simulink model "pwm_motor"  (R2021b)
settings: Solver=VariableStepAuto  StartTime=0.0  StopTime=1  RelTol=1e-3
undefined symbols (not defined in the file or in its folder): J, km, L, R, Vmax
libraries: simulink x2
settings Model: Creator=cirie  LastModifiedBy=cirie

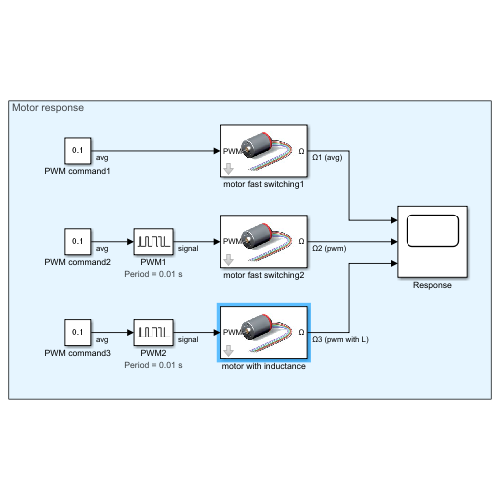
[thumbnail: Simulink's stored preview of the top-level diagram]
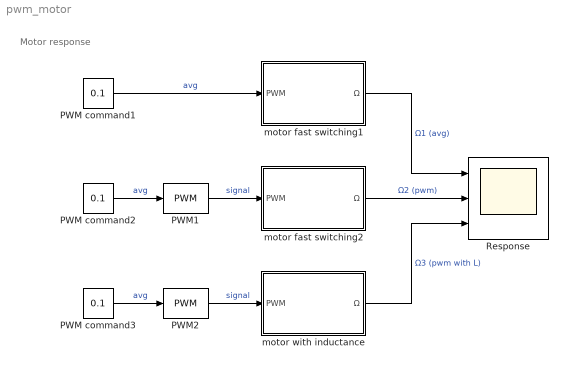
== system pwm_motor ==
  note: Motor response
  PWM command1 : Constant  Value=0.1
  PWM command2 : Constant  Value=0.1
  PWM command3 : Constant  Value=0.1
  PWM1 : simulink/Discontinuities/PWM  DisableCoverage=on  Period=0.01  DisallowZeroDutyCycle=off  RunAtFixedTimeIntervals=off  SampleTime=0.01
      settings: AttributesFormatString=Period = %<Period> s
  PWM2 : simulink/Discontinuities/PWM  DisableCoverage=on  Period=0.01  DisallowZeroDutyCycle=off  RunAtFixedTimeIntervals=off  SampleTime=0.01
      settings: AttributesFormatString=Period = %<Period> s
  Response : Scope  NumInputPorts=3
  motor fast switching1 : Subsystem  mask(DC Motor){J=J, km=km, R=R, Vmax=Vmax}
      mask prompts: J "Inertia, J [kgm^2]"; km "Motor constant, km [V*s/rad]"; R "Resistance, R [Ohm]"; Vmax "Maximum Voltage, Vmax [V]"
      mask help:
      | Circuit Dynamics:   PWM*Vmax == I*R + km*Ω
      | Rotor Dynamics:     J*dΩ/dt == km*I
      mask Display: image('$imagefile'); % Use "Edit Image" on toolstrip to change.
  motor fast switching2 : Subsystem  mask(DC Motor){J=J, km=km, R=R, Vmax=Vmax}
      mask prompts: J "Inertia, J [kgm^2]"; km "Motor constant, km [V*s/rad]"; R "Resistance, R [Ohm]"; Vmax "Maximum Voltage, Vmax [V]"
      mask help:
      | Circuit Dynamics:   PWM*Vmax == I*R + km*Ω
      | Rotor Dynamics:     J*dΩ/dt == km*I
      mask Display: image('$imagefile'); % Use "Edit Image" on toolstrip to change.
  motor with inductance : Subsystem  mask(DC Motor){J=J, km=km, R=R, L=L, Vmax=Vmax}
      mask prompts: J "Inertia, J [kgm^2]"; km "Motor constant, km [V*s/rad]"; R "Resistance, R [Ohm]"; L "Inductance, L [H]"; Vmax "Maximum Voltage, Vmax [V]"
      mask help:
      | Circuit Dynamics:   PWM*Vmax == I*R + km*Ω
      | Rotor Dynamics:     J*dΩ/dt == km*I
      mask Display: image('$imagefile'); % Use "Edit Image" on toolstrip to change.
  wires:
  motor with inductance/1(Ω) -> Response/3  "Ω3 (pwm with L)"
  motor fast switching2/1(Ω) -> Response/2  "Ω2 (pwm)"
  motor fast switching1/1(Ω) -> Response/1  "Ω1 (avg)"
  PWM command1/1 -> motor fast switching1/1(PWM)  "avg"
  PWM command2/1 -> PWM1/1  "avg"
  PWM1/1 -> motor fast switching2/1(PWM)  "signal"
  PWM command3/1 -> PWM2/1  "avg"
  PWM2/1 -> motor with inductance/1(PWM)  "signal"

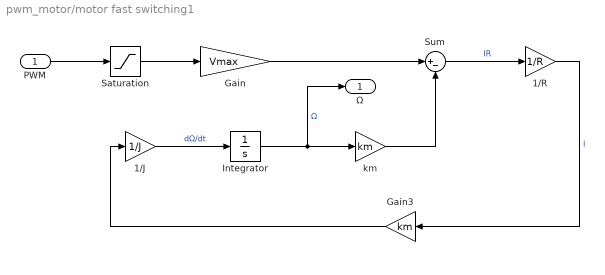
== system pwm_motor/motor fast switching1 ==
  PWM : Inport
  1/J : Gain  Gain=1/J
  1/R : Gain  Gain=1/R
  Gain : Gain  Gain=Vmax
  Gain3 : Gain  Gain=km
  Integrator : Integrator
  Saturation : Saturate  UpperLimit=1  LowerLimit=-1
  Sum : Sum  Inputs=|+-
  km : Gain  Gain=km
  Ω : Outport
  wires:
  1/J/1 -> Integrator/1  "dΩ/dt"
  Sum/1 -> 1/R/1  "IR"
  Integrator/1 -> Ω/1, km/1  "Ω"
  Gain3/1 -> 1/J/1
  km/1 -> Sum/2
  1/R/1 -> Gain3/1  "I"
  PWM/1 -> Saturation/1
  Gain/1 -> Sum/1
  Saturation/1 -> Gain/1

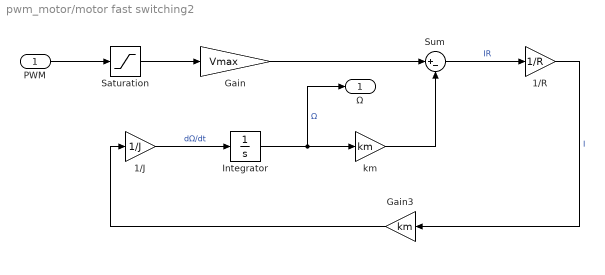
== system pwm_motor/motor fast switching2 ==
  PWM : Inport
  1/J : Gain  Gain=1/J
  1/R : Gain  Gain=1/R
  Gain : Gain  Gain=Vmax
  Gain3 : Gain  Gain=km
  Integrator : Integrator
  Saturation : Saturate  UpperLimit=1  LowerLimit=-1
  Sum : Sum  Inputs=|+-
  km : Gain  Gain=km
  Ω : Outport
  wires:
  Saturation/1 -> Gain/1
  Gain/1 -> Sum/1
  PWM/1 -> Saturation/1
  1/R/1 -> Gain3/1  "I"
  km/1 -> Sum/2
  Gain3/1 -> 1/J/1
  Integrator/1 -> km/1, Ω/1  "Ω"
  Sum/1 -> 1/R/1  "IR"
  1/J/1 -> Integrator/1  "dΩ/dt"

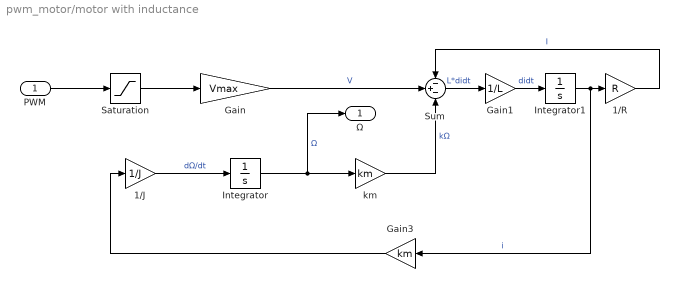
== system pwm_motor/motor with inductance ==
  PWM : Inport
  1/J : Gain  Gain=1/J
  1/R : Gain  Gain=R
  Gain : Gain  Gain=Vmax
  Gain1 : Gain  Gain=1/L
  Gain3 : Gain  Gain=km
  Integrator : Integrator
  Integrator1 : Integrator
  Saturation : Saturate  UpperLimit=1  LowerLimit=-1
  Sum : Sum  Inputs=-+-
  km : Gain  Gain=km
  Ω : Outport
  wires:
  1/J/1 -> Integrator/1  "dΩ/dt"
  Integrator1/1 -> Gain3/1, 1/R/1  "i"
  Integrator/1 -> Ω/1, km/1  "Ω"
  Gain3/1 -> 1/J/1
  km/1 -> Sum/3  "kΩ"
  1/R/1 -> Sum/1  "I"
  PWM/1 -> Saturation/1
  Gain/1 -> Sum/2  "V"
  Saturation/1 -> Gain/1
  Sum/1 -> Gain1/1  "L*didt"
  Gain1/1 -> Integrator1/1  "didt"
